simulink model "Practica1_MSF1_MAT"  (R2024b)
settings: Solver=VariableStepAuto  StartTime=0.0  StopTime=10.0  RelTol=1e-3
libraries: slpidlib x1, simulink x1
settings Model: Creator=ASUS  LastModifiedBy=Angel Torales
settings DataIOCC: SaveOutput=off  SignalLogging=off  DSMLogging=off  ReturnWorkspaceOutputs=off  TimeSaveName=t
settings DebuggingCC: AlgebraicLoopMsg=none  ArtificialAlgebraicLoopMsg=none  MaxConsecutiveZCsMsg=none  OperatingPointInterfaceChecksumMismatchMsg=none

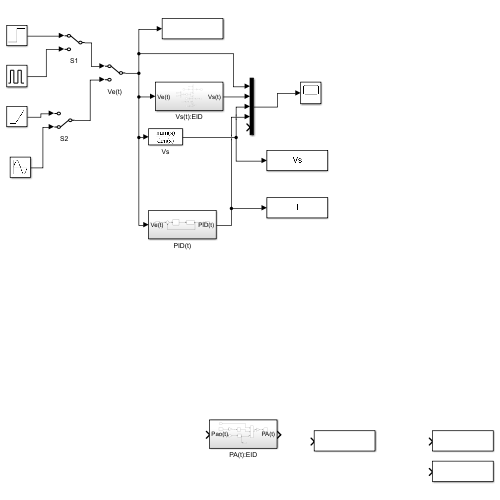
[thumbnail: Simulink's stored preview of the top-level diagram]
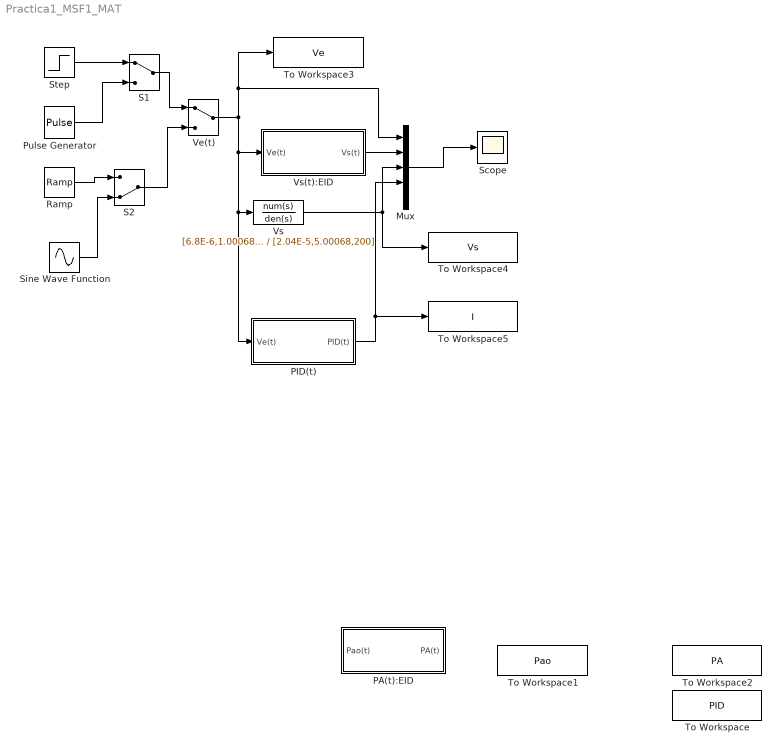
== system Practica1_MSF1_MAT ==
  Mux : Mux  Inputs=5
  PA(t):EID : Subsystem
  PID(t) : Subsystem
  Pulse Generator : DiscretePulseGenerator  PulseType=Time based  Period=10  PulseWidth=10  PhaseDelay=1
  Ramp : simulink/Sources/Ramp  slope=1/10  start=0  InitialOutput=0
  S1 : ManualSwitch
  S2 : ManualSwitch  CurrentSetting=0
  Scope : Scope
  Sine Wave Function : Sin  Frequency=pi/2
  Step : Step  Time=0  Before=1  SampleTime=0
  To Workspace : ToWorkspace  VariableName=PID  SampleTime=-1
  To Workspace1 : ToWorkspace  VariableName=Pao  SampleTime=-1
  To Workspace2 : ToWorkspace  VariableName=PA  SampleTime=-1
  To Workspace3 : ToWorkspace  VariableName=Ve  SampleTime=-1
  To Workspace4 : ToWorkspace  VariableName=Vs  SampleTime=-1
  To Workspace5 : ToWorkspace  VariableName=I  SampleTime=-1
  Ve(t) : ManualSwitch
  Vs : TransferFcn  Numerator=[6.8E-6,1.00068,100]  Denominator=[2.04E-5,5.00068,200]
  Vs(t):EID : Subsystem
  wires:
  Vs(t):EID/1(Vs(t)) -> Mux/2
  Mux/1 -> Scope/1
  Vs/1 -> To Workspace4/1, Mux/3
  Step/1 -> S1/1
  Pulse Generator/1 -> S1/2
  S1/1 -> Ve(t)/1
  Ve(t)/1 -> To Workspace3/1, Mux/1, Vs(t):EID/1(Ve(t)), PID(t)/1(Ve(t)), Vs/1
  Ramp/1 -> S2/1
  Sine Wave Function/1 -> S2/2
  S2/1 -> Ve(t)/2
  PID(t)/1(PID(t)) -> Mux/4, To Workspace5/1

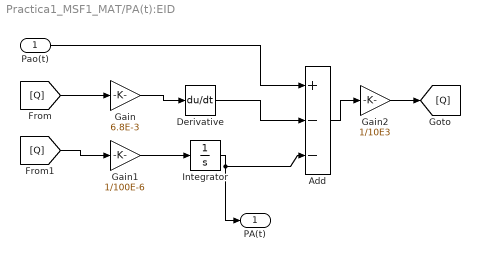
== system Practica1_MSF1_MAT/PA(t):EID ==
  Pao(t) : Inport
  Add : Sum  Inputs=+--
  Derivative : Derivative
  Gain : Gain  Gain=6.8E-3
  Gain1 : Gain  Gain=1/100E-6
  Gain2 : Gain  Gain=1/10E3
  Integrator : Integrator
  PA(t) : Outport
  wires:
  Pao(t)/1 -> Add/1
  [Q] -> Gain/1
  Gain/1 -> Derivative/1
  Derivative/1 -> Add/2
  [Q] -> Gain1/1
  Gain1/1 -> Integrator/1
  Integrator/1 -> PA(t)/1, Add/3
  Add/1 -> Gain2/1
  Gain2/1 -> [Q]

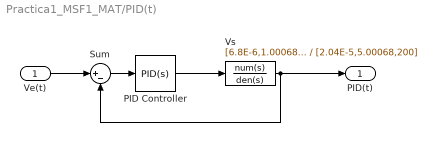
== system Practica1_MSF1_MAT/PID(t) ==
  Ve(t) : Inport
  PID Controller : slpidlib/PID Controller  Controller=PID  Form=Parallel  TimeDomain=Continuous-time  UseExternalTs=off  SampleTime=-1  IntegratorMethod=Forward Euler  FilterMethod=Forward Euler  ControllerParametersSource=internal  P=0  I=3989613.63863787  UseKiTs=off  D=0  UseExternalDerivativeSource=off  N=100  UseFilter=on  TunerSelectOption=Transfer Function Based (PID Tuner App)  InitialConditionSource=internal  InitialConditionForIntegrator=0  InitialConditionForFilter=0  DifferentiatorICPrevScaledInput=0  ExternalReset=none  TrackingMode=off  Kt=1  LimitOutput=off  SatLimitsSource=internal  UpperSaturationLimit=inf  LowerSaturationLimit=-inf  LinearizeAsGain=on  AntiWindupMode=none  Kb=1  LimitIntegrator=off  UpperIntegratorSaturationLimit=inf  LowerIntegratorSaturationLimit=-inf  POutMin=[]  POutMax=[]  IOutMin=[]  IOutMax=[]  DOutMin=[]  DOutMax=[]  NOutMin=[]  NOutMax=[]  SumOutMin=[]  SumOutMax=[]  SaturationOutMin=[]  SaturationOutMax=[]  PParamMin=[]  PParamMax=[]  IParamMin=[]  IParamMax=[]  DParamMin=[]  DParamMax=[]  NParamMin=[]  NParamMax=[]  KbParamMin=[]  KbParamMax=[]  KtParamMin=[]  KtParamMax=[]  KbOutMin=[]  KbOutMax=[]  KtOutMin=[]  KtOutMax=[]  IntegratorOutMin=[]  IntegratorOutMax=[]  FilterOutMin=[]  FilterOutMax=[]  SumI1OutMin=[]  SumI1OutMax=[]  SumI2OutMin=[]  SumI2OutMax=[]  SumI3OutMin=[]  SumI3OutMax=[]  SumI4OutMin=[]  SumI4OutMax=[]  SumDOutMin=[]  SumDOutMax=[]  DifferentiatorOutMin=[]  DifferentiatorOutMax=[]  FilterDiffOutCoefMin=[]  FilterDiffOutCoefMax=[]  ReciprocalOutMin=[]  ReciprocalOutMax=[]  SumDenOutMin=[]  SumDenOutMax=[]  SumNumOutMin=[]  SumNumOutMax=[]  DivideOutMin=[]  DivideOutMax=[]  UdiffTsProdOutMin=[]  UdiffTsProdOutMax=[]  NTsProdOutMin=[]  NTsProdOutMax=[]  UintegralTsProdOutMin=[]  UintegralTsProdOutMax=[]  UngainTsProdOutMin=[]  UngainTsProdOutMax=[]  ClampingZeroOutDataTypeStr=Inherit: Inherit via back propagation  ClampingZeroOutMin=[]  ClampingZeroOutMax=[]  FilterDenConstantOutDataTypeStr=Inherit: Inherit via back propagation  FilterDenConstantOutMin=[]  FilterDenConstantOutMax=[]  PCopyOutDataTypeStr=Inherit: Inherit via back propagation  PCopyOutMin=[]  PCopyOutMax=[]  NCopyOutDataTypeStr=Inherit: Inherit via back propagation  NCopyOutMin=[]  NCopyOutMax=[]  IntegratorContinuousStateAttributes=''  IntegratorStateMustResolveToSignalObject=off  IntegratorRTWStateStorageClass=Auto  FilterContinuousStateAttributes=''  FilterStateMustResolveToSignalObject=off  FilterRTWStateStorageClass=Auto  ParallelPVariant=InternalParameters  IdealPVariant=Disabled  IVariant=InternalParameters  DVariant=InternalParameters  IntegratorVariant=Continuous  SatVariant=Disabled  AWVariant=Passthrough  PCopyVariant=Disabled  TRVariant=Disabled  FdbkBlocksVariant=Forward  IdealPFdbkVariant=Disabled  SatFdbkVariant=Disabled  DerivativeFilterVariant=ContFilter  NVariant=InternalParameters  NCopyVariant=Disabled  FilterICVariant=InternalICsFilter  IntegratorICVariant=InternalICs  ExternalResetVariant=Disabled  TRSumVariant=Passthrough  SumFdbkVariant=Disabled  SumVariant=Sum_PID  TsampFilterVariant=InternalTs  TsampNgainVariant=Passthrough  TsampIntegralVariant=Disabled_SignalSpec  ExternalSaturationOutDataTypeStr=Inherit: Same as second input  DerivativeSourceVariant=ErrorSignal  PreIntVariant=InternalPreInt
  Sum : Sum  Inputs=|+-
  Vs : TransferFcn  Numerator=[6.8E-6,1.00068,100]  Denominator=[2.04E-5,5.00068,200]
  PID(t) : Outport
  wires:
  Sum/1 -> PID Controller/1
  PID Controller/1 -> Vs/1
  Vs/1 -> Sum/2, PID(t)/1
  Ve(t)/1 -> Sum/1

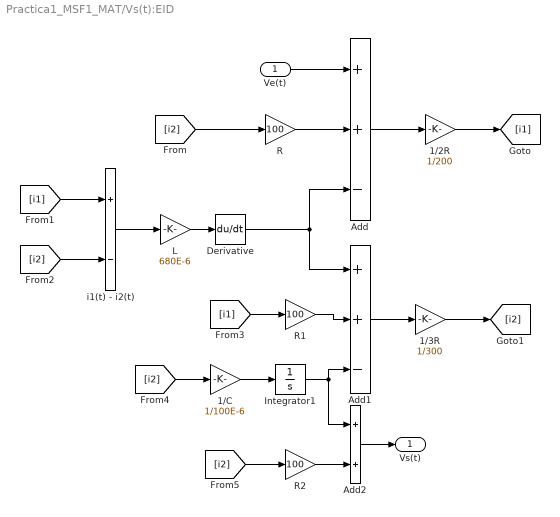
== system Practica1_MSF1_MAT/Vs(t):EID ==
  Ve(t) : Inport
  1/2R : Gain  Gain=1/200
  1/3R : Gain  Gain=1/300
  1/C : Gain  Gain=1/100E-6
  Add : Sum  Inputs=++-
  Add1 : Sum  Inputs=++-
  Add2 : Sum
  Derivative : Derivative
  Integrator1 : Integrator
  L : Gain  Gain=680E-6
  R : Gain  Gain=100
  R1 : Gain  Gain=100
  R2 : Gain  Gain=100
  i1(t) - i2(t) : Sum  Inputs=+-
  Vs(t) : Outport
  wires:
  Ve(t)/1 -> Add/1
  Derivative/1 -> Add1/1, Add/3
  Add/1 -> 1/2R/1
  1/2R/1 -> [i1]
  [i2] -> R/1
  R/1 -> Add/2
  L/1 -> Derivative/1
  [i1] -> i1(t) - i2(t)/1
  [i2] -> i1(t) - i2(t)/2
  i1(t) - i2(t)/1 -> L/1
  1/C/1 -> Integrator1/1
  Integrator1/1 -> Add2/1, Add1/3
  [i2] -> 1/C/1
  [i2] -> R2/1
  R2/1 -> Add2/2
  Add2/1 -> Vs(t)/1
  [i1] -> R1/1
  R1/1 -> Add1/2
  1/3R/1 -> [i2]
  Add1/1 -> 1/3R/1
